simulink model "sfediticon"  (Simulink 6.0)
settings: Solver=FixedStepDiscrete  StartTime=0.0  StopTime=inf  RelTol=1e-3
CloseFcn:
  | sf_edit_icon('kill');
settings Model: CovMetricSettings=dcmtr  Creator=The MathWorks Inc.  LastModifiedBy=batserve  ExtModeTrigMode=oneshot  ExtModeArmWhenConnect=off  ExtModeAutoUpdateStatusClock=off
settings DataIOCC: LimitDataPoints=off  SaveOutput=off  SaveTime=off
settings OptimizationCC: BooleanDataType=off
settings DebuggingCC: CheckExecutionContextPreStartOutputMsg=on  CheckExecutionContextRuntimeOutputMsg=on  SolverPrmCheckMsg=none
settings HardwareCC: TargetUnknown=on

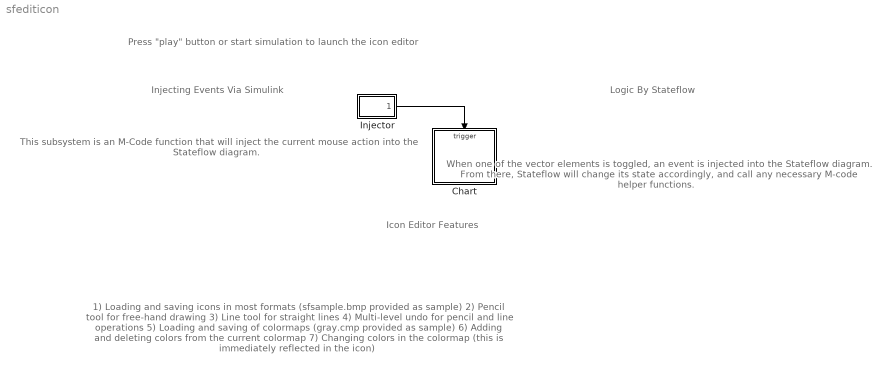
== system sfediticon ==
  note: This subsystem is an M-Code
      | function that will inject the
      | current mouse action into the
      | Stateflow diagram.
  note: Injecting Events
      | Via Simulink
  note: When one of the vector elements
      | is toggled, an event is injected
      | into the Stateflow diagram.
      | From there, Stateflow will
      | change its state accordingly,
      | and call any necessary M-code
      | helper functions.
  note: Logic By Stateflow
  note: 1) Loading and saving icons in most formats
      |      (sfsample.bmp provided as sample)
      | 2) Pencil tool for free-hand drawing
      | 3) Line tool for straight lines
      | 4) Multi-level undo for pencil and line operations
      | 5) Loading and saving of colormaps
      |      (gray.cmp provided as sample)
      | 6) Adding and deleting colors from the current
      |      colormap
      | 7) Changing colors in the colormap
      |     (this is immediately reflected in the icon)
  note: Icon Editor Features
  note: Press "play" button or start simulation to launch the icon editor
  Chart : Stateflow chart  PropExecContextAcrossSSBoundary=on
  Injector : Subsystem  PropExecContextAcrossSSBoundary=on
  wires:
  Injector/1(Event) -> Chart/Trigger

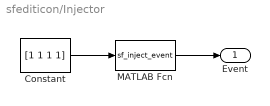
== system sfediticon/Injector ==
  Constant : Constant  Value=[1 1 1 1]
  MATLAB Fcn : MATLABFcn  MATLABFcn=sf_inject_event
  Event : Outport
  wires:
  MATLAB Fcn/1 -> Event/1
  Constant/1 -> MATLAB Fcn/1

== stateflow chart Chart ==
  settings: executeAtInitialization=1
  state ToolBar [parallel]
    state Released
    state Locked
      en:
      ml.sf_edit_icon...
      ('status', 'Tool locked');
    state Pressed
      en:
      pressedIcon = focusedIcon;
      press(pressedIcon,1);
      ex: press(pressedIcon,0);
    state icon_operation(icon) [function]
      (default) -> (junction 26)
      (junction 26) -> (junction 27)
      (junction 26) -> (junction 28) : [icon == OPEN_ICON] {ml.sf_edit_icon('open');}
      (junction 33) -> (junction 32) : [icon == SAVE_MAP_ICON] {ml.sf_edit_icon('save_map');}
      (junction 27) -> (junction 29) : [icon == SAVE_ICON] {ml.sf_edit_icon('save_as');}
      (junction 27) -> (junction 30)
      (junction 30) -> (junction 31) : [icon == OPEN_MAP_ICON] {ml.sf_edit_icon('open_map');}
      (junction 33) -> (junction 34)
      (junction 34) -> (junction 70) : [icon == UNDO_ICON] {ml.sf_edit_icon('undo');}
      (junction 30) -> (junction 33)
    state None
      pressedIcon = 0;
      ml.sf_edit_icon('status', 'Select a tool');
      ml.sf_edit_icon('normal_cursor');
    state press(icon,sp) [function]
      (junction 42) -> (junction 25)
      (junction 35) -> (junction 37) : [icon == OPEN_MAP_ICON] {ml.sf_edit_icon('press',sp,'open_map');}
      (junction 38) -> (junction 44) : [icon == SAVE_MAP_ICON] {ml.sf_edit_icon('press', sp, 'save_map');}
      (junction 40) -> (junction 36) : [icon == SAVE_ICON] {ml.sf_edit_icon('press', sp, 'save_as');}
      (junction 40) -> (junction 35)
      (junction 35) -> (junction 38)
      (junction 46) -> (junction 43) : [icon == UNDO_ICON] {ml.sf_edit_icon('press',sp,'undo');}
      (junction 42) -> (junction 58) : [icon == LINE_ICON] {ml.sf_edit_icon('press',sp,'line');}
      (junction 46) -> (junction 42)
      (junction 38) -> (junction 46)
      (junction 61) -> (junction 40)
      (default) -> (junction 61)
      (junction 61) -> (junction 39) : [icon == OPEN_ICON] {ml.sf_edit_icon('press', sp, 'open');}
      (junction 25) -> (junction 69) : [icon == PENCIL_ICON] {ml.sf_edit_icon('press',sp,'pencil');}
    ToolBar.None -> Pressed : NBD [in(Focus.Toolbar)]
    Released -> Pressed : BM [pressedIcon == focusedIcon]
    Pressed -> Released : BM [pressedIcon != focusedIcon]
    (junction 62) -> ToolBar.None : {icon_operation(pressedIcon);}
    Released -> ToolBar.None : BU
    (junction 62) -> Locked : [(pressedIcon == LINE_ICON)]...
        | {ml.sf_edit_icon('line_cursor');}
    Locked -> Pressed : NBD[in(Focus.Toolbar)]
    (default) -> ToolBar.None
    (junction 62) -> Locked : [(pressedIcon == PENCIL_ICON)]...
        | {ml.sf_edit_icon('pencil_cursor');}
    Pressed -> (junction 62) : BU
  state Focus [parallel]
    state Palette
      state None
      state Swatch
      (junction 45) -> Focus.Palette.None
      (junction 45) -> Swatch : [ml.sf_edit_icon...
          | ('over_color_swatch')]
    state Icon
    state Canvas
    state None
    state Toolbar
      en: set_focusedIcon();
      du: set_focusedIcon();
      ex: focusedIcon = 0;
    state set_focusedIcon() [function]
      (default) -> (junction 48)
      (junction 48) -> (junction 49) : [ml.sf_edit_icon('over_open_tool')] ...
          | {focusedIcon = OPEN_ICON;}
      (junction 48) -> (junction 50)
      (junction 50) -> (junction 51) : [ml.sf_edit_icon('over_saveas_tool')]...
          | {focusedIcon = SAVE_ICON;}
      (junction 50) -> (junction 52)
      (junction 52) -> (junction 53) : [ml.sf_edit_icon('over_openmap_tool')]...
          |  {focusedIcon = OPEN_MAP_ICON;}
      (junction 52) -> (junction 55)
      (junction 55) -> (junction 54) : [ml.sf_edit_icon('over_savemap_tool')] ...
          | {focusedIcon = SAVE_MAP_ICON;}
      (junction 55) -> (junction 56)
      (junction 56) -> (junction 57) : [ml.sf_edit_icon('over_undo_tool')]...
          |  {focusedIcon = UNDO_ICON;}
      (junction 65) -> (junction 47) : {focusedIcon = 0;}
      (junction 56) -> (junction 63)
      (junction 63) -> (junction 64) : [ml.sf_edit_icon('over_line_tool')]...
          |  {focusedIcon = LINE_ICON;}
      (junction 63) -> (junction 65)
      (junction 65) -> (junction 66) : [ml.sf_edit_icon('over_pencil_tool')]...
          |  {focusedIcon = PENCIL_ICON;}
    (default) -> Focus.None
    (junction 41) -> Icon : [ml.sf_edit_icon('over_icon')]
    (junction 41) -> Canvas : [ml.sf_edit_icon('over_canvas')]
    (junction 41) -> Focus.None
    Focus -> (junction 41) : BM
    (junction 41) -> (junction 45) : [ml.sf_edit_icon('over_palette')]
    (junction 41) -> (junction 68) : [ml.sf_edit_icon('over_toolbar')]
    (junction 68) -> Toolbar
    (junction 68) -> (junction 59) : [in(Toolbar)]
  state Main [parallel]
    state FGColorSelect
      en: ml.sf_edit_icon('cache_color');
      ex: ml.sf_edit_icon('fgcolor');
    state PencilDraw
      en: ml.sf_edit_icon('draw_point');
      du: ml.sf_edit_icon('draw_point');
      ex:  ml.sf_edit_icon('commit');
    state Idle
    state LineDraw
      en: ml.sf_edit_icon('anchor_line');
      du: ml.sf_edit_icon('render_line');
      ex:  ml.sf_edit_icon('commit');
    Idle -> (junction 67) : ABD[in(Focus.Palette.Swatch)]
        | {ml.sf_edit_icon('show_color_menu');}
    Idle -> (junction 60) : NBD[in(ToolBar.Locked)&&...
        |          in(Focus.Canvas)]
    Idle -> FGColorSelect : NBD[in(Focus.Palette.Swatch)]
    (junction 60) -> PencilDraw : [pressedIcon == PENCIL_ICON]
    (default) -> Idle : {ml.sf_edit_icon('create');}
    (junction 60) -> LineDraw : [pressedIcon == LINE_ICON]
    Main -> Idle : BU
  state Note: [group]
    Make sure "Focus" comes before "Tool".
    The Tool state depends on up-to-date
    information about the Focus.
  data: icon function_input double; Canvas local double; Icon local double; Palette local double; icon function_input double; sp function_input double; LINE_ICON constant int32 =1; OPEN_ICON constant int32 =2; OPEN_MAP_ICON constant int32 =3; PENCIL_ICON constant int32 =4; SAVE_MAP_ICON constant int32 =5; UNDO_ICON constant int32 =6; pressedIcon local int32; focusedIcon local int32; SAVE_ICON constant int32 =7
  events: BM input EITHER_EDGE_EVENT; NBD input EITHER_EDGE_EVENT; BU input EITHER_EDGE_EVENT; ABD input EITHER_EDGE_EVENT
